simulink model "Boeing737Sample_updatedCopy_sb_12_7_2014"  (R2013b)
settings: Solver=ode23tb  StartTime=0.0  StopTime=10  RelTol=1e-3
InitFcn:
  | load('loss_coeff_mixing_junction.mat')
  | %load('defaultMSSN.mat')
  | load('SampleOutput.mat')
  | load('HydProp.mat')
  | load('HydraulicLoad.mat')
  | 
  | %load('mission_short.mat')
values from neighbouring files (symbols this model uses):
  FuelBurn = [0 0 0 0 0 0 0 0 0 0 0 0 ... (18249 elements, 1x18249)]    [Benchmark_data1.mat]
undefined symbols (not defined in the file or in its folder): ailerons, B_737, elevator, F1, F2, HUGHES_TREITLER, landing_gear, PN_70147, rudder, thrust_rev
libraries: PowerFlowLib x97, simulink x15
(part 8 of 8)

== system Boeing737Sample_updatedCopy_sb_12_7_2014/ECS & FOS /FOHX Right Wing/HX_Calcs/Fluid 2 Heat Transfer Calculation ==
  note: NTU calculation
  note: Secondary Fluid heat transfer coefficient
  note: It calculates the outlet temperature and enthalpy.
  Inputs : Inport
  1-D Lookup Table : Lookup_n-D  NumberOfTableDimensions=1  BreakpointsForDimension1=F2.T  Table=F2.cp_T  RndMeth=Simplest  InputSameDT=on
  1-D Lookup Table1 : Lookup_n-D  NumberOfTableDimensions=1  BreakpointsForDimension1=F2.T  Table=F2.H  RndMeth=Simplest  InputSameDT=on
  1-D Lookup Table2 : Lookup_n-D  NumberOfTableDimensions=1  BreakpointsForDimension1=F2.T  Table=F2.H  RndMeth=Simplest  InputSameDT=on
  1-D Lookup Table3 : Lookup_n-D  NumberOfTableDimensions=1  BreakpointsForDimension1=F2.T  Table=F2.H  RndMeth=Simplest  InputSameDT=on
  Bus Selector : BusSelector  OutputSignals=mdot2_in,T2_in,P2_in
  Constant : Constant  Value=0
  Constant10 : Constant  Value=A2_c
  Constant2 : Constant  Value=N2
  Constant4 : Constant
  Constant8 : Constant  Value=N2
  Constant9 : Constant  Value=A2_s*2
  Fcn6 : Fcn  Expr=u(2) + (u(1)-u(2))*u(3)
  Gain1 : Gain  Gain=-1
  Gain3 : Gain  Gain=-1
  HTC Calc : Subsystem
  Math Function3 : Math  SaturateOnIntegerOverflow=on
  Mux4 : Mux  Inputs=3
  Product2 : Product  Inputs=***//  RndMeth=Zero
  Product6 : Product  Inputs=***/  RndMeth=Zero
  Subtract2 : Sum  Inputs=+-
  Terminator : Terminator
  kJ/kg to J/kg : Gain  Gain=1000
  h_out : Outport
  T_out : Outport  Port=2
  q_h : Outport  Port=3
  wires:
  [T_out] -> 1-D Lookup Table3/1
  [T_in] -> 1-D Lookup Table2/1
  1-D Lookup Table2/1 -> Subtract2/1
  1-D Lookup Table3/1 -> Subtract2/2
  1-D Lookup Table1/1 -> h_out/1
  Product6/1 -> Gain1/1
  Constant4/1 -> Product6/2
  [mdot_in] -> Product6/1
  Subtract2/1 -> Product6/3
  Fcn6/1 -> [T_out], T_out/1, 1-D Lookup Table1/1  "T_out"
  Mux4/1 -> Fcn6/1
  [e2NTU1] -> Mux4/3
  Constant/1 -> Mux4/2
  Gain1/1 -> q_h/1
  Constant2/1 -> Product6/4
  Product2/1 -> Gain3/1  "NTU"
  Constant9/1 -> Product2/2
  [alpha] -> Product2/1
  Constant8/1 -> Product2/3
  HTC Calc/1(alpha_a) -> [alpha]
  [T_in] -> HTC Calc/3(T_a)
  Constant10/1 -> HTC Calc/2(A_ca)
  [mdot_in] -> HTC Calc/1(mdot_a)
  [T_in] -> 1-D Lookup Table/1
  1-D Lookup Table/1 -> kJ/kg to J/kg/1
  Inputs/1 -> Bus Selector/1
  Bus Selector/1 -> [mdot_in]  "<mdot2_in>"
  Bus Selector/2 -> [T_in]  "<T2_in>"
  Bus Selector/3 -> Terminator/1  "<P2_in>"
  Math Function3/1 -> [e2NTU1]
  Gain3/1 -> Math Function3/1
  [mdot_in] -> Product2/4
  [cp] -> Product2/5
  [T_in] -> Mux4/1
  kJ/kg to J/kg/1 -> [cp]

== system Boeing737Sample_updatedCopy_sb_12_7_2014/ECS & FOS /FOHX Right Wing/HX_Calcs/Input Processing ==
  Inputs : Inport
  Bus Creator : BusCreator  Inputs=6
  Bus Selector : BusSelector  OutputSignals=mdot1_in,P1_in,T1_in,mdot2_in,P2_in,T2_in
  Processed_Inputs : Outport
  wires:
  Bus Selector/1 -> Bus Creator/1  "<mdot1_in>"
  Bus Selector/2 -> Bus Creator/2  "<P1_in>"
  Bus Selector/3 -> Bus Creator/3  "<T1_in>"
  Bus Selector/4 -> Bus Creator/4  "<mdot2_in>"
  Bus Selector/5 -> Bus Creator/5  "<P2_in>"
  Bus Selector/6 -> Bus Creator/6  "<T2_in>"
  Inputs/1 -> Bus Selector/1  "Inputs"
  Bus Creator/1 -> Processed_Inputs/1

== system Boeing737Sample_updatedCopy_sb_12_7_2014/ECS & FOS /FOHX Left Wing/HX_Calcs/Fluid 1 Heat Transfer Calculation/HTC Calc ==
  note: Calculation of secondary fluid heat transfer coefficient using the Longo correlation
  mdot_a : Inport
  A_ca : Inport  Port=2
  T_a : Inport  Port=3
  Constant1 : Constant  Value=alpha1
  Terminator : Terminator
  Terminator1 : Terminator
  Terminator2 : Terminator
  alpha_a : Outport
  wires:
  T_a/1 -> Terminator2/1
  A_ca/1 -> Terminator1/1
  mdot_a/1 -> Terminator/1
  Constant1/1 -> alpha_a/1

== system Boeing737Sample_updatedCopy_sb_12_7_2014/ECS & FOS /FOHX Left Wing/HX_Calcs/Fluid 2 Heat Transfer Calculation/HTC Calc ==
  note: Calculation of secondary fluid heat transfer coefficient using the Longo correlation
  mdot_a : Inport
  A_ca : Inport  Port=2
  T_a : Inport  Port=3
  Constant1 : Constant  Value=alpha2
  Terminator : Terminator
  Terminator1 : Terminator
  Terminator2 : Terminator
  alpha_a : Outport
  wires:
  T_a/1 -> Terminator2/1
  A_ca/1 -> Terminator1/1
  mdot_a/1 -> Terminator/1
  Constant1/1 -> alpha_a/1

== system Boeing737Sample_updatedCopy_sb_12_7_2014/ECS & FOS /FOHX Right Wing/HX_Calcs/Fluid 1 Heat Transfer Calculation/HTC Calc ==
  note: Calculation of secondary fluid heat transfer coefficient using the Longo correlation
  mdot_a : Inport
  A_ca : Inport  Port=2
  T_a : Inport  Port=3
  Constant1 : Constant  Value=alpha1
  Terminator : Terminator
  Terminator1 : Terminator
  Terminator2 : Terminator
  alpha_a : Outport
  wires:
  Constant1/1 -> alpha_a/1
  mdot_a/1 -> Terminator/1
  A_ca/1 -> Terminator1/1
  T_a/1 -> Terminator2/1

== system Boeing737Sample_updatedCopy_sb_12_7_2014/ECS & FOS /FOHX Right Wing/HX_Calcs/Fluid 2 Heat Transfer Calculation/HTC Calc ==
  note: Calculation of secondary fluid heat transfer coefficient using the Longo correlation
  mdot_a : Inport
  A_ca : Inport  Port=2
  T_a : Inport  Port=3
  Constant1 : Constant  Value=alpha2
  Terminator : Terminator
  Terminator1 : Terminator
  Terminator2 : Terminator
  alpha_a : Outport
  wires:
  Constant1/1 -> alpha_a/1
  mdot_a/1 -> Terminator/1
  A_ca/1 -> Terminator1/1
  T_a/1 -> Terminator2/1
